simulink model "slowdown"  (R2014a)
settings: Solver=ode3  StartTime=0.0  StopTime=Inf  FixedStep=0.01  RelTol=1e-3
undefined symbols (not defined in the file or in its folder): now
libraries: simulink x3
settings Model: Creator=eruffaldi  LastModifiedBy=eruffaldi

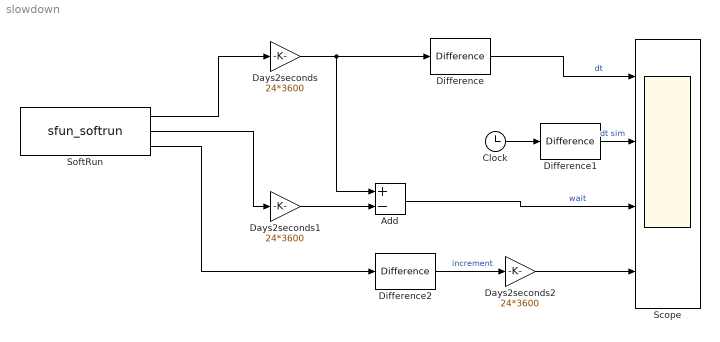
== system slowdown ==
  Add : Sum  Inputs=+-
  Clock : Clock
  Days2seconds : Gain  Gain=24*3600
  Days2seconds1 : Gain  Gain=24*3600
  Days2seconds2 : Gain  Gain=24*3600
  Difference : simulink/Discrete/Difference  ICPrevInput=now*24*3600  InputProcessing=Inherited  OutMin=[]  OutMax=[]  OutDataType=fixdt(1, 16)  OutScaling=2^-10  DoSatur=off
  Difference1 : simulink/Discrete/Difference  ICPrevInput=0.0  InputProcessing=Inherited  OutMin=[]  OutMax=[]  OutDataType=fixdt(1, 16)  OutScaling=2^-10  DoSatur=off
  Difference2 : simulink/Discrete/Difference  ICPrevInput=now  InputProcessing=Inherited  OutMin=[]  OutMax=[]  OutDataType=fixdt(1, 16)  OutScaling=2^-10  DoSatur=off
  Scope : Scope  NumInputPorts=4
      settings: YMin=-3.46945e-18~0~0~0  YMax=0.08~0.0125~900~0.045
  SoftRun : M-S-Function  FunctionName=sfun_softrun  Parameters=step  mask(Keyboard Input){step=0.01}
      mask help: Keyboard Input
      mask Display:
      | fprintf('Soft Run');
      | port_label('output',1,'time');
      | port_label('output',2,'pre');
      | port_label('output',3,'next');
  wires:
  SoftRun/1 -> Days2seconds/1
  Clock/1 -> Difference1/1
  Difference1/1 -> Scope/2  "dt sim"
  Difference/1 -> Scope/1  "dt"
  SoftRun/2 -> Days2seconds1/1
  Days2seconds/1 -> Add/1, Difference/1
  SoftRun/3 -> Difference2/1
  Difference2/1 -> Days2seconds2/1  "increment"
  Days2seconds1/1 -> Add/2
  Add/1 -> Scope/3  "wait"
  Days2seconds2/1 -> Scope/4
